simulink model "full_3omni_ctrl_sim_and_exp_with_bbb"  (R2019b)
settings: Solver=ode3  StartTime=0.0  StopTime=40  FixedStep=0.01  RelTol=1e-3  EnableMultiTasking=on
libraries: bbblueCommlib x24, simulink x10, bbblueSensorLib x4, xpcutilitieslib x3, xpcrtudplib x2, slrtlib x1
(part 1 of 2)
settings Model: SimulationMode=external  ExtModeTrigDuration=100  Creator=Sarot PC  LastModifiedBy=ONLY-GOD
settings SolverCC: PositivePriorityOrder=on
settings DataIOCC: SaveFormat=StructureWithTime
settings OptimizationCC: BlockReduction=off  EnhancedBackFolding=on  PassReuseOutputArgsAs=Individual arguments  ZeroExternalMemoryAtStartup=off  ZeroInternalMemoryAtStartup=off  MaxStackSize=64  OptimizeBlockOrder=speed  DifferentSizesBufferReuse=on  OptimizationCustomize=off  EfficientTunableParamExpr=on
settings DebuggingCC: ParameterTunabilityLossMsg=error  SFExecutionAtInitializationDiag=none  ArithmeticOperatorsInVariantConditions=warning
settings HardwareCC: ProdBitPerPointer=32  ProdBitPerSizeT=32  ProdBitPerPtrDiffT=32  ProdLargestAtomicInteger=Long  ProdLargestAtomicFloat=Double  ProdWordSize=32  ProdHWDeviceType=ARM Compatible->ARM Cortex
settings SFSimCC: MATLABDynamicMemAlloc=off  CustomCodeUndefinedFunction=UseInterfaceOnly
settings RTWCC: SystemTargetFile=ert.tlc  HardwareBoard=BeagleBone Blue  TLCOptions="-aInlineSetEventsForThisBaseRateFcn=TLC_FALSE -aSuppressMultiTaskScheduler=TLC_FALSE  -aRateBasedStepFcn=0"  TemplateMakefile=ert_default_tmf  GenerateReport=on  Toolchain=GNU GCC BeagleBone Blue  IncludeHyperlinkInReport=on  LaunchReport=on  GenerateTraceInfo=on  GenerateTraceReport=on  GenerateTraceReportSl=on  GenerateTraceReportSf=on  GenerateTraceReportEml=on
settings CodeAppCC: ForceParamTrailComments=on  IgnoreCustomStorageClasses=off  OperatorAnnotations=on  SimulinkDataObjDesc=on  SFDataObjDesc=on  InsertBlockDesc=on
settings ERTTargetCC: SupportContinuousTime=on  SupportVariableSizeSignals=on

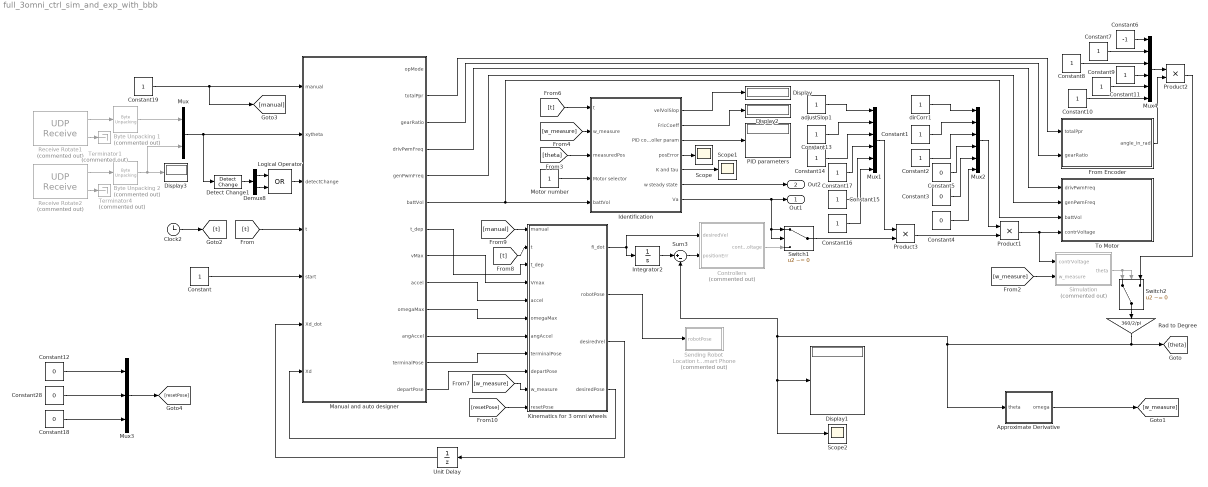
== system full_3omni_ctrl_sim_and_exp_with_bbb ==
  Approximate Derivative : Subsystem
  Byte Unpacking 1 : xpcutilitieslib/Byte Unpacking   Commented=on  MaskUnpackedDataTypes={'double'}  MaskUnpackedDataSizes={[1]}  MaskAlignment=1
      settings: SourceProductName=Simulink Real-Time  SourceProductBaseCode=XP
  Byte Unpacking 2 : xpcutilitieslib/Byte Unpacking   Commented=on  MaskUnpackedDataTypes={'double'}  MaskUnpackedDataSizes={[1]}  MaskAlignment=1
      settings: SourceProductName=Simulink Real-Time  SourceProductBaseCode=XP
  Clock2 : Clock
  Constant{,1..2,7..11,13..17,19} (14 alike) : Constant
  Constant{3..5,12,18,28} (6 alike) : Constant  Value=0
  Constant6 : Constant  Value=-1
  Controllers : Subsystem  Commented=on
  Demux8 : Demux  Outputs=2
  Detect Change1 : simulink/Logic and Bit Operations/Detect Change  vinit=0  OutDataTypeStr=boolean
  Display{,1..3} (4 alike) : Display
  From Encoder : Subsystem
  Identification : Subsystem
  Integrator2 : Integrator  InitialCondition=zeros(6,1)
  Kinematics for 3 omni wheels : Subsystem
  Logical Operator : Logic  Operator=OR  AllPortsSameDT=off  OutDataTypeStr=boolean
  Manual and auto designer : Stateflow chart  TreatAsAtomicUnit=on
  Motor number : Constant
  Mux : Mux  Inputs=2
  Mux1 : Mux  Inputs=6
  Mux2 : Mux  Inputs=6
  Mux3 : Mux  Inputs=3
  Mux4 : Mux  Inputs=6
  PID parameters : Display
  Product1 : Product
  Product2 : Product
  Product3 : Product
  Rad to Degree : Gain  Gain=360/2/pi
  Receive Rotate1 : xpcrtudplib/UDP Receive  Commented=on  ipAddressVal=Use host-target connection  localPort=2501  rcvWidth=8  rcvFmAny=off  fmAddress=192.168.88.233  rcvMulticast=off  multicastAddress={}  maxUDPQueue=8  sampleTime=-1
      settings: SourceProductName=Simulink Real-Time
  Receive Rotate2 : xpcrtudplib/UDP Receive  Commented=on  ipAddressVal=Use host-target connection  localPort=2502  rcvWidth=8  rcvFmAny=off  fmAddress=192.168.88.233  rcvMulticast=off  multicastAddress={}  maxUDPQueue=8  sampleTime=-1
      settings: SourceProductName=Simulink Real-Time
  Scope : Scope
  Scope1 : Scope
  Scope2 : Scope
  Sending Robot Location to Smart Phone : Subsystem  Commented=on
  Simulation : Subsystem  Commented=on
  Sum3 : Sum  Inputs=|+-
  Switch1 : Switch  Criteria=u2 ~= 0
  Switch2 : Switch  Criteria=u2 ~= 0
  Terminator1 : Terminator  Commented=on
  Terminator4 : Terminator  Commented=on
  To Motor : Subsystem
  Unit Delay : UnitDelay  InitialCondition=[0;0;0]  SampleTime=-1  HasFrameUpgradeWarning=on
  adjustSlop1 : Constant
  dirCorr1 : Constant
  Out1 : Outport
  Out2 : Outport  Port=2
  wires:
  Constant2/1 -> Mux2/3
  dirCorr1/1 -> Mux2/1
  Constant1/1 -> Mux2/2
  Mux2/1 -> Product1/1
  Product1/1 -> Simulation/1(contrVoltage), To Motor/4(contrVoltage)
  Product3/1 -> Product1/2
  Constant5/1 -> Mux2/4
  Constant3/1 -> Mux2/5
  Constant4/1 -> Mux2/6
  Constant10/1 -> Mux4/6
  Constant6/1 -> Mux4/1
  Constant7/1 -> Mux4/2
  Mux4/1 -> Product2/1
  Constant11/1 -> Mux4/4
  Constant9/1 -> Mux4/5
  Constant8/1 -> Mux4/3
  From Encoder/1(angle_in_rad) -> Product2/2
  Product2/1 -> Switch2/3
  Constant16/1 -> Mux1/6
  Constant15/1 -> Mux1/5
  Constant17/1 -> Mux1/4
  Mux1/1 -> Product3/1
  Constant13/1 -> Mux1/2
  adjustSlop1/1 -> Mux1/1
  Constant14/1 -> Mux1/3
  Switch1/1 -> Product3/2
  Manual and auto designer/2(totalPpr) -> From Encoder/1(totalPpr)
  Manual and auto designer/3(gearRatio) -> From Encoder/2(gearRatio)
  Simulation/1(theta) -> Switch2/2, Switch2/1
  Controllers/1(contrVoltage) -> Switch1/3
  Sum3/1 -> Controllers/2(positionErr)
  Identification/7(Va) -> Out1/1, Switch1/2, Switch1/1
  [t] -> Identification/1(t)
  [w_measure] -> Identification/2(w_measure)
  [theta] -> Identification/3(measuredPos)
  Identification/1(velVolSlop) -> Display/1
  Identification/3(PID controller param) -> PID parameters/1
  Identification/6(w steady state) -> Out2/1
  Identification/4(posError) -> Scope/1
  Identification/5(K and tau) -> Scope1/1
  Motor number/1 -> Identification/4(Motor selector)
  Integrator2/1 -> Sum3/1
  Kinematics for 3 omni wheels/1(fi_dot) -> Integrator2/1, Controllers/1(desiredVel)
  Manual and auto designer/4(drivPwmFreq) -> To Motor/1(drivPwmFreq)
  Manual and auto designer/5(genPwmFreq) -> To Motor/2(genPwmFreq)
  Manual and auto designer/6(battVol) -> To Motor/3(battVol), Identification/5(battVol)
  Identification/2(FricCoeff) -> Display2/1
  [w_measure] -> Simulation/2(w_measure)
  Demux8/2 -> Logical Operator/2
  Logical Operator/1 -> Manual and auto designer/3(detectChange)
  Mux/1 -> Detect Change1/1, Manual and auto designer/2(xytheta)
  Detect Change1/1 -> Demux8/1
  Kinematics for 3 omni wheels/4(desiredPose) -> Manual and auto designer/7(Xd)
  [t] -> Manual and auto designer/4(t)
  Constant/1 -> Manual and auto designer/5(start)
  Demux8/1 -> Logical Operator/1
  Constant19/1 -> [manual], Manual and auto designer/1(manual)
  Clock2/1 -> [t]
  [t] -> Kinematics for 3 omni wheels/2(t)
  Kinematics for 3 omni wheels/2(robotPose) -> Sending Robot Location to Smart Phone/1(robotPose)
  [w_measure] -> Kinematics for 3 omni wheels/10(w_measure)
  Kinematics for 3 omni wheels/3(desiredVel) -> Unit Delay/1
  Manual and auto designer/13(departPose) -> Kinematics for 3 omni wheels/9(departPose)
  Manual and auto designer/12(terminalPose) -> Kinematics for 3 omni wheels/8(terminalPose)
  Manual and auto designer/10(omegaMax) -> Kinematics for 3 omni wheels/6(omegaMax)
  Manual and auto designer/11(angAccel) -> Kinematics for 3 omni wheels/7(angAccel)
  Manual and auto designer/9(accel) -> Kinematics for 3 omni wheels/5(accel)
  Manual and auto designer/8(vMax) -> Kinematics for 3 omni wheels/4(Vmax)
  Manual and auto designer/7(t_dep) -> Kinematics for 3 omni wheels/3(t_dep)
  [manual] -> Kinematics for 3 omni wheels/1(manual)
  Unit Delay/1 -> Manual and auto designer/6(Xd_dot)
  Constant12/1 -> Mux3/1
  Constant28/1 -> Mux3/2
  Constant18/1 -> Mux3/3
  Mux3/1 -> [resetPose]
  [resetPose] -> Kinematics for 3 omni wheels/11(resetPose)
  Receive Rotate2/1 -> Byte Unpacking 2/1
  Receive Rotate1/2 -> Terminator1/1
  Byte Unpacking 1/1 -> Mux/1
  Receive Rotate2/2 -> Terminator4/1
  Receive Rotate1/1 -> Byte Unpacking 1/1
  Byte Unpacking 2/1 -> Mux/2, Display3/1
  Rad to Degree/1 -> [theta], Sum3/2, Scope2/1, Display1/1, Approximate Derivative/1(theta)
  Approximate Derivative/1(omega) -> [w_measure]
  Switch2/1 -> Rad to Degree/1

== system full_3omni_ctrl_sim_and_exp_with_bbb/Approximate Derivative ==
  theta : Inport
  Demux7 : Demux  Outputs=6
  Mux3 : Mux  Inputs=6
  Transfer Fcn{,1..5} (6 alike) : TransferFcn  Numerator=[1 0]  Denominator=[0.04 1]
  omega : Outport
  wires:
  Transfer Fcn1/1 -> Mux3/2
  Demux7/5 -> Transfer Fcn4/1
  Transfer Fcn3/1 -> Mux3/4
  Demux7/3 -> Transfer Fcn2/1
  Demux7/6 -> Transfer Fcn5/1
  Transfer Fcn2/1 -> Mux3/3
  Transfer Fcn/1 -> Mux3/1
  Transfer Fcn5/1 -> Mux3/6
  Demux7/4 -> Transfer Fcn3/1
  Mux3/1 -> omega/1
  Transfer Fcn4/1 -> Mux3/5
  Demux7/1 -> Transfer Fcn/1
  Demux7/2 -> Transfer Fcn1/1
  theta/1 -> Demux7/1

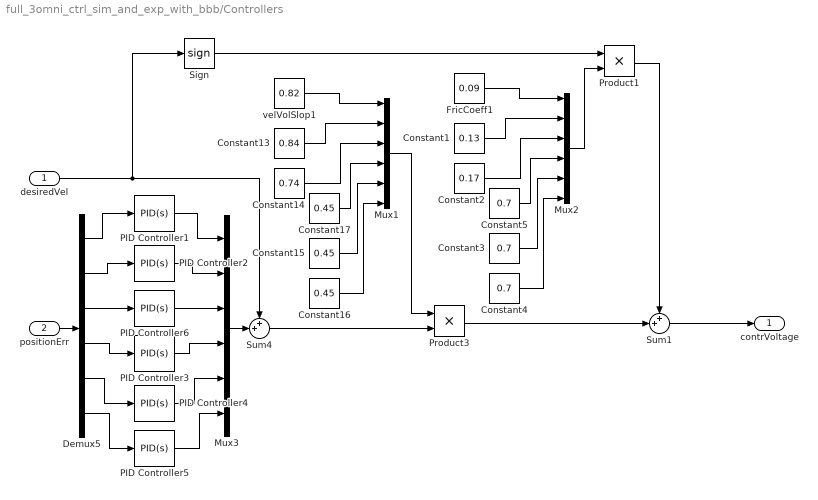
== system full_3omni_ctrl_sim_and_exp_with_bbb/Controllers ==
  desiredVel : Inport
  positionErr : Inport  Port=2
  Constant1 : Constant  Value=0.13
  Constant13 : Constant  Value=0.84
  Constant14 : Constant  Value=0.74
  Constant15 : Constant  Value=0.45
  Constant16 : Constant  Value=0.45
  Constant17 : Constant  Value=0.45
  Constant2 : Constant  Value=0.17
  Constant3 : Constant  Value=0.7
  Constant4 : Constant  Value=0.7
  Constant5 : Constant  Value=0.7
  Demux5 : Demux  Outputs=6
  FricCoeff1 : Constant  Value=0.09
  Mux1 : Mux  Inputs=6
  Mux2 : Mux  Inputs=6
  Mux3 : Mux  Inputs=6
  "PID Controller1 " : simulink/Continuous/PID Controller  Controller=PID  Form=Parallel  TimeDomain=Continuous-time  SampleTime=-1  IntegratorMethod=Forward Euler  FilterMethod=Forward Euler  ControllerParametersSource=internal  P=45/0.82  I=0  D=2.9/0.82  UseFilter=on  N=100  TunerSelectOption=Transfer Function Based (PID Tuner App)  InitialConditionSource=internal  InitialConditionForIntegrator=0  InitialConditionForFilter=0  DifferentiatorICPrevScaledInput=0  ExternalReset=none  TrackingMode=off  Kt=1  LimitOutput=off  UpperSaturationLimit=inf  LowerSaturationLimit=-inf  LinearizeAsGain=on  AntiWindupMode=none  Kb=1  POutMin=[]  POutMax=[]  IOutMin=[]  IOutMax=[]  DOutMin=[]  DOutMax=[]  NOutMin=[]  NOutMax=[]  SumOutMin=[]  SumOutMax=[]  SaturationOutMin=[]  SaturationOutMax=[]  PParamMin=[]  PParamMax=[]  IParamMin=[]  IParamMax=[]  DParamMin=[]  DParamMax=[]  NParamMin=[]  NParamMax=[]  KbParamMin=[]  KbParamMax=[]  KtParamMin=[]  KtParamMax=[]  KbOutMin=[]  KbOutMax=[]  KtOutMin=[]  KtOutMax=[]  IntegratorOutMin=[]  IntegratorOutMax=[]  FilterOutMin=[]  FilterOutMax=[]  SumI1OutMin=[]  SumI1OutMax=[]  SumI2OutMin=[]  SumI2OutMax=[]  SumI3OutMin=[]  SumI3OutMax=[]  SumI4OutMin=[]  SumI4OutMax=[]  SumDOutMin=[]  SumDOutMax=[]  DifferentiatorOutMin=[]  DifferentiatorOutMax=[]  FilterDiffOutCoefMin=[]  FilterDiffOutCoefMax=[]  ReciprocalOutMin=[]  ReciprocalOutMax=[]  SumDenOutMin=[]  SumDenOutMax=[]  SumNumOutMin=[]  SumNumOutMax=[]  DivideOutMin=[]  DivideOutMax=[]  IntegratorContinuousStateAttributes=''  IntegratorStateMustResolveToSignalObject=off  IntegratorRTWStateStorageClass=Auto  FilterContinuousStateAttributes=''  FilterStateMustResolveToSignalObject=off  FilterRTWStateStorageClass=Auto  ParallelPVariant=InternalParameters  IdealPVariant=Disabled  IVariant=InternalParameters  DVariant=InternalParameters  IntegratorVariant=Continuous  SatVariant=Disabled  AWVariant=Passthrough  PCopyVariant=Disabled  TRVariant=Disabled  FdbkBlocksVariant=Forward  IdealPFdbkVariant=Disabled  SatFdbkVariant=Disabled  DerivativeFilterVariant=ContFilter  NVariant=InternalParameters  NCopyVariant=Disabled  FilterICVariant=InternalICsFilter  IntegratorICVariant=InternalICs  ExternalResetVariant=Disabled  TRSumVariant=Passthrough  SumFdbkVariant=Disabled  SumVariant=Sum_PID
  PID Controller2 : simulink/Continuous/PID Controller  Controller=PID  Form=Parallel  TimeDomain=Continuous-time  SampleTime=-1  IntegratorMethod=Forward Euler  FilterMethod=Forward Euler  ControllerParametersSource=internal  P=45/0.84  I=0  D=2.96/0.84  UseFilter=on  N=100  TunerSelectOption=Transfer Function Based (PID Tuner App)  InitialConditionSource=internal  InitialConditionForIntegrator=0  InitialConditionForFilter=0  DifferentiatorICPrevScaledInput=0  ExternalReset=none  TrackingMode=off  Kt=1  LimitOutput=off  UpperSaturationLimit=inf  LowerSaturationLimit=-inf  LinearizeAsGain=on  AntiWindupMode=none  Kb=1  POutMin=[]  POutMax=[]  IOutMin=[]  IOutMax=[]  DOutMin=[]  DOutMax=[]  NOutMin=[]  NOutMax=[]  SumOutMin=[]  SumOutMax=[]  SaturationOutMin=[]  SaturationOutMax=[]  PParamMin=[]  PParamMax=[]  IParamMin=[]  IParamMax=[]  DParamMin=[]  DParamMax=[]  NParamMin=[]  NParamMax=[]  KbParamMin=[]  KbParamMax=[]  KtParamMin=[]  KtParamMax=[]  KbOutMin=[]  KbOutMax=[]  KtOutMin=[]  KtOutMax=[]  IntegratorOutMin=[]  IntegratorOutMax=[]  FilterOutMin=[]  FilterOutMax=[]  SumI1OutMin=[]  SumI1OutMax=[]  SumI2OutMin=[]  SumI2OutMax=[]  SumI3OutMin=[]  SumI3OutMax=[]  SumI4OutMin=[]  SumI4OutMax=[]  SumDOutMin=[]  SumDOutMax=[]  DifferentiatorOutMin=[]  DifferentiatorOutMax=[]  FilterDiffOutCoefMin=[]  FilterDiffOutCoefMax=[]  ReciprocalOutMin=[]  ReciprocalOutMax=[]  SumDenOutMin=[]  SumDenOutMax=[]  SumNumOutMin=[]  SumNumOutMax=[]  DivideOutMin=[]  DivideOutMax=[]  IntegratorContinuousStateAttributes=''  IntegratorStateMustResolveToSignalObject=off  IntegratorRTWStateStorageClass=Auto  FilterContinuousStateAttributes=''  FilterStateMustResolveToSignalObject=off  FilterRTWStateStorageClass=Auto  ParallelPVariant=InternalParameters  IdealPVariant=Disabled  IVariant=InternalParameters  DVariant=InternalParameters  IntegratorVariant=Continuous  SatVariant=Disabled  AWVariant=Passthrough  PCopyVariant=Disabled  TRVariant=Disabled  FdbkBlocksVariant=Forward  IdealPFdbkVariant=Disabled  SatFdbkVariant=Disabled  DerivativeFilterVariant=ContFilter  NVariant=InternalParameters  NCopyVariant=Disabled  FilterICVariant=InternalICsFilter  IntegratorICVariant=InternalICs  ExternalResetVariant=Disabled  TRSumVariant=Passthrough  SumFdbkVariant=Disabled  SumVariant=Sum_PID
  PID Controller3 : simulink/Continuous/PID Controller  Controller=PID  Form=Parallel  TimeDomain=Continuous-time  SampleTime=-1  IntegratorMethod=Forward Euler  FilterMethod=Forward Euler  ControllerParametersSource=internal  P=10  I=0  D=3  UseFilter=on  N=100  TunerSelectOption=Transfer Function Based (PID Tuner App)  InitialConditionSource=internal  InitialConditionForIntegrator=0  InitialConditionForFilter=0  DifferentiatorICPrevScaledInput=0  ExternalReset=none  TrackingMode=off  Kt=1  LimitOutput=off  UpperSaturationLimit=inf  LowerSaturationLimit=-inf  LinearizeAsGain=on  AntiWindupMode=none  Kb=1  POutMin=[]  POutMax=[]  IOutMin=[]  IOutMax=[]  DOutMin=[]  DOutMax=[]  NOutMin=[]  NOutMax=[]  SumOutMin=[]  SumOutMax=[]  SaturationOutMin=[]  SaturationOutMax=[]  PParamMin=[]  PParamMax=[]  IParamMin=[]  IParamMax=[]  DParamMin=[]  DParamMax=[]  NParamMin=[]  NParamMax=[]  KbParamMin=[]  KbParamMax=[]  KtParamMin=[]  KtParamMax=[]  KbOutMin=[]  KbOutMax=[]  KtOutMin=[]  KtOutMax=[]  IntegratorOutMin=[]  IntegratorOutMax=[]  FilterOutMin=[]  FilterOutMax=[]  SumI1OutMin=[]  SumI1OutMax=[]  SumI2OutMin=[]  SumI2OutMax=[]  SumI3OutMin=[]  SumI3OutMax=[]  SumI4OutMin=[]  SumI4OutMax=[]  SumDOutMin=[]  SumDOutMax=[]  DifferentiatorOutMin=[]  DifferentiatorOutMax=[]  FilterDiffOutCoefMin=[]  FilterDiffOutCoefMax=[]  ReciprocalOutMin=[]  ReciprocalOutMax=[]  SumDenOutMin=[]  SumDenOutMax=[]  SumNumOutMin=[]  SumNumOutMax=[]  DivideOutMin=[]  DivideOutMax=[]  IntegratorContinuousStateAttributes=''  IntegratorStateMustResolveToSignalObject=off  IntegratorRTWStateStorageClass=Auto  FilterContinuousStateAttributes=''  FilterStateMustResolveToSignalObject=off  FilterRTWStateStorageClass=Auto  ParallelPVariant=InternalParameters  IdealPVariant=Disabled  IVariant=InternalParameters  DVariant=InternalParameters  IntegratorVariant=Continuous  SatVariant=Disabled  AWVariant=Passthrough  PCopyVariant=Disabled  TRVariant=Disabled  FdbkBlocksVariant=Forward  IdealPFdbkVariant=Disabled  SatFdbkVariant=Disabled  DerivativeFilterVariant=ContFilter  NVariant=InternalParameters  NCopyVariant=Disabled  FilterICVariant=InternalICsFilter  IntegratorICVariant=InternalICs  ExternalResetVariant=Disabled  TRSumVariant=Passthrough  SumFdbkVariant=Disabled  SumVariant=Sum_PID
  PID Controller4 : simulink/Continuous/PID Controller  Controller=PID  Form=Parallel  TimeDomain=Continuous-time  SampleTime=-1  IntegratorMethod=Forward Euler  FilterMethod=Forward Euler  ControllerParametersSource=internal  P=10  I=0  D=3  UseFilter=on  N=100  TunerSelectOption=Transfer Function Based (PID Tuner App)  InitialConditionSource=internal  InitialConditionForIntegrator=0  InitialConditionForFilter=0  DifferentiatorICPrevScaledInput=0  ExternalReset=none  TrackingMode=off  Kt=1  LimitOutput=off  UpperSaturationLimit=inf  LowerSaturationLimit=-inf  LinearizeAsGain=on  AntiWindupMode=none  Kb=1  POutMin=[]  POutMax=[]  IOutMin=[]  IOutMax=[]  DOutMin=[]  DOutMax=[]  NOutMin=[]  NOutMax=[]  SumOutMin=[]  SumOutMax=[]  SaturationOutMin=[]  SaturationOutMax=[]  PParamMin=[]  PParamMax=[]  IParamMin=[]  IParamMax=[]  DParamMin=[]  DParamMax=[]  NParamMin=[]  NParamMax=[]  KbParamMin=[]  KbParamMax=[]  KtParamMin=[]  KtParamMax=[]  KbOutMin=[]  KbOutMax=[]  KtOutMin=[]  KtOutMax=[]  IntegratorOutMin=[]  IntegratorOutMax=[]  FilterOutMin=[]  FilterOutMax=[]  SumI1OutMin=[]  SumI1OutMax=[]  SumI2OutMin=[]  SumI2OutMax=[]  SumI3OutMin=[]  SumI3OutMax=[]  SumI4OutMin=[]  SumI4OutMax=[]  SumDOutMin=[]  SumDOutMax=[]  DifferentiatorOutMin=[]  DifferentiatorOutMax=[]  FilterDiffOutCoefMin=[]  FilterDiffOutCoefMax=[]  ReciprocalOutMin=[]  ReciprocalOutMax=[]  SumDenOutMin=[]  SumDenOutMax=[]  SumNumOutMin=[]  SumNumOutMax=[]  DivideOutMin=[]  DivideOutMax=[]  IntegratorContinuousStateAttributes=''  IntegratorStateMustResolveToSignalObject=off  IntegratorRTWStateStorageClass=Auto  FilterContinuousStateAttributes=''  FilterStateMustResolveToSignalObject=off  FilterRTWStateStorageClass=Auto  ParallelPVariant=InternalParameters  IdealPVariant=Disabled  IVariant=InternalParameters  DVariant=InternalParameters  IntegratorVariant=Continuous  SatVariant=Disabled  AWVariant=Passthrough  PCopyVariant=Disabled  TRVariant=Disabled  FdbkBlocksVariant=Forward  IdealPFdbkVariant=Disabled  SatFdbkVariant=Disabled  DerivativeFilterVariant=ContFilter  NVariant=InternalParameters  NCopyVariant=Disabled  FilterICVariant=InternalICsFilter  IntegratorICVariant=InternalICs  ExternalResetVariant=Disabled  TRSumVariant=Passthrough  SumFdbkVariant=Disabled  SumVariant=Sum_PID
  PID Controller5 : simulink/Continuous/PID Controller  Controller=PID  Form=Parallel  TimeDomain=Continuous-time  SampleTime=-1  IntegratorMethod=Forward Euler  FilterMethod=Forward Euler  ControllerParametersSource=internal  P=10  I=0  D=3  UseFilter=on  N=100  TunerSelectOption=Transfer Function Based (PID Tuner App)  InitialConditionSource=internal  InitialConditionForIntegrator=0  InitialConditionForFilter=0  DifferentiatorICPrevScaledInput=0  ExternalReset=none  TrackingMode=off  Kt=1  LimitOutput=off  UpperSaturationLimit=inf  LowerSaturationLimit=-inf  LinearizeAsGain=on  AntiWindupMode=none  Kb=1  POutMin=[]  POutMax=[]  IOutMin=[]  IOutMax=[]  DOutMin=[]  DOutMax=[]  NOutMin=[]  NOutMax=[]  SumOutMin=[]  SumOutMax=[]  SaturationOutMin=[]  SaturationOutMax=[]  PParamMin=[]  PParamMax=[]  IParamMin=[]  IParamMax=[]  DParamMin=[]  DParamMax=[]  NParamMin=[]  NParamMax=[]  KbParamMin=[]  KbParamMax=[]  KtParamMin=[]  KtParamMax=[]  KbOutMin=[]  KbOutMax=[]  KtOutMin=[]  KtOutMax=[]  IntegratorOutMin=[]  IntegratorOutMax=[]  FilterOutMin=[]  FilterOutMax=[]  SumI1OutMin=[]  SumI1OutMax=[]  SumI2OutMin=[]  SumI2OutMax=[]  SumI3OutMin=[]  SumI3OutMax=[]  SumI4OutMin=[]  SumI4OutMax=[]  SumDOutMin=[]  SumDOutMax=[]  DifferentiatorOutMin=[]  DifferentiatorOutMax=[]  FilterDiffOutCoefMin=[]  FilterDiffOutCoefMax=[]  ReciprocalOutMin=[]  ReciprocalOutMax=[]  SumDenOutMin=[]  SumDenOutMax=[]  SumNumOutMin=[]  SumNumOutMax=[]  DivideOutMin=[]  DivideOutMax=[]  IntegratorContinuousStateAttributes=''  IntegratorStateMustResolveToSignalObject=off  IntegratorRTWStateStorageClass=Auto  FilterContinuousStateAttributes=''  FilterStateMustResolveToSignalObject=off  FilterRTWStateStorageClass=Auto  ParallelPVariant=InternalParameters  IdealPVariant=Disabled  IVariant=InternalParameters  DVariant=InternalParameters  IntegratorVariant=Continuous  SatVariant=Disabled  AWVariant=Passthrough  PCopyVariant=Disabled  TRVariant=Disabled  FdbkBlocksVariant=Forward  IdealPFdbkVariant=Disabled  SatFdbkVariant=Disabled  DerivativeFilterVariant=ContFilter  NVariant=InternalParameters  NCopyVariant=Disabled  FilterICVariant=InternalICsFilter  IntegratorICVariant=InternalICs  ExternalResetVariant=Disabled  TRSumVariant=Passthrough  SumFdbkVariant=Disabled  SumVariant=Sum_PID
  PID Controller6 : simulink/Continuous/PID Controller  Controller=PID  Form=Parallel  TimeDomain=Continuous-time  SampleTime=-1  IntegratorMethod=Forward Euler  FilterMethod=Forward Euler  ControllerParametersSource=internal  P=45/0.74  I=0  D=2.59/0.74  UseFilter=on  N=100  TunerSelectOption=Transfer Function Based (PID Tuner App)  InitialConditionSource=internal  InitialConditionForIntegrator=0  InitialConditionForFilter=0  DifferentiatorICPrevScaledInput=0  ExternalReset=none  TrackingMode=off  Kt=1  LimitOutput=off  UpperSaturationLimit=inf  LowerSaturationLimit=-inf  LinearizeAsGain=on  AntiWindupMode=none  Kb=1  POutMin=[]  POutMax=[]  IOutMin=[]  IOutMax=[]  DOutMin=[]  DOutMax=[]  NOutMin=[]  NOutMax=[]  SumOutMin=[]  SumOutMax=[]  SaturationOutMin=[]  SaturationOutMax=[]  PParamMin=[]  PParamMax=[]  IParamMin=[]  IParamMax=[]  DParamMin=[]  DParamMax=[]  NParamMin=[]  NParamMax=[]  KbParamMin=[]  KbParamMax=[]  KtParamMin=[]  KtParamMax=[]  KbOutMin=[]  KbOutMax=[]  KtOutMin=[]  KtOutMax=[]  IntegratorOutMin=[]  IntegratorOutMax=[]  FilterOutMin=[]  FilterOutMax=[]  SumI1OutMin=[]  SumI1OutMax=[]  SumI2OutMin=[]  SumI2OutMax=[]  SumI3OutMin=[]  SumI3OutMax=[]  SumI4OutMin=[]  SumI4OutMax=[]  SumDOutMin=[]  SumDOutMax=[]  DifferentiatorOutMin=[]  DifferentiatorOutMax=[]  FilterDiffOutCoefMin=[]  FilterDiffOutCoefMax=[]  ReciprocalOutMin=[]  ReciprocalOutMax=[]  SumDenOutMin=[]  SumDenOutMax=[]  SumNumOutMin=[]  SumNumOutMax=[]  DivideOutMin=[]  DivideOutMax=[]  IntegratorContinuousStateAttributes=''  IntegratorStateMustResolveToSignalObject=off  IntegratorRTWStateStorageClass=Auto  FilterContinuousStateAttributes=''  FilterStateMustResolveToSignalObject=off  FilterRTWStateStorageClass=Auto  ParallelPVariant=InternalParameters  IdealPVariant=Disabled  IVariant=InternalParameters  DVariant=InternalParameters  IntegratorVariant=Continuous  SatVariant=Disabled  AWVariant=Passthrough  PCopyVariant=Disabled  TRVariant=Disabled  FdbkBlocksVariant=Forward  IdealPFdbkVariant=Disabled  SatFdbkVariant=Disabled  DerivativeFilterVariant=ContFilter  NVariant=InternalParameters  NCopyVariant=Disabled  FilterICVariant=InternalICsFilter  IntegratorICVariant=InternalICs  ExternalResetVariant=Disabled  TRSumVariant=Passthrough  SumFdbkVariant=Disabled  SumVariant=Sum_PID
  Product1 : Product
  Product3 : Product
  Sign : Signum
  Sum1 : Sum  Inputs=++|
  Sum4 : Sum  Inputs=++|
  velVolSlop1 : Constant  Value=0.82
  contrVoltage : Outport
  wires:
  PID Controller2/1 -> Mux3/2
  Demux5/3 -> PID Controller6/1
  Demux5/1 -> "PID Controller1 "/1
  PID Controller6/1 -> Mux3/3
  "PID Controller1 "/1 -> Mux3/1
  positionErr/1 -> Demux5/1
  Demux5/2 -> PID Controller2/1
  Demux5/4 -> PID Controller3/1
  Demux5/5 -> PID Controller4/1
  Demux5/6 -> PID Controller5/1
  PID Controller3/1 -> Mux3/4
  PID Controller4/1 -> Mux3/5
  PID Controller5/1 -> Mux3/6
  Constant16/1 -> Mux1/6
  Constant15/1 -> Mux1/5
  Constant14/1 -> Mux1/3
  Constant13/1 -> Mux1/2
  velVolSlop1/1 -> Mux1/1
  Mux1/1 -> Product3/1
  Constant17/1 -> Mux1/4
  Sum1/1 -> contrVoltage/1
  Mux3/1 -> Sum4/2
  Sum4/1 -> Product3/2
  desiredVel/1 -> Sign/1, Sum4/1
  Product3/1 -> Sum1/2
  Constant2/1 -> Mux2/3
  Constant5/1 -> Mux2/4
  FricCoeff1/1 -> Mux2/1
  Constant4/1 -> Mux2/6
  Constant3/1 -> Mux2/5
  Constant1/1 -> Mux2/2
  Sign/1 -> Product1/1
  Mux2/1 -> Product1/2
  Product1/1 -> Sum1/1

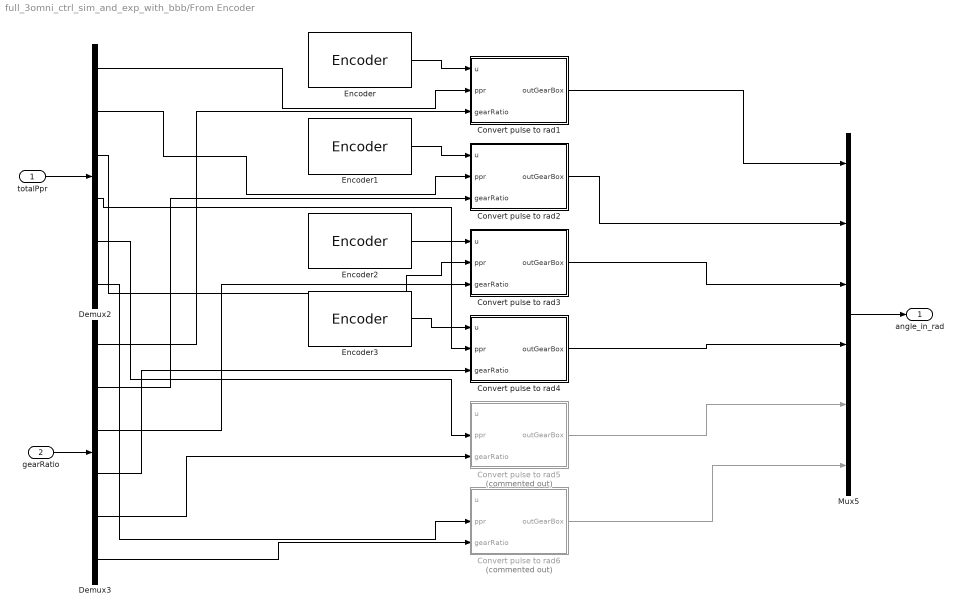
== system full_3omni_ctrl_sim_and_exp_with_bbb/From Encoder ==
  totalPpr : Inport
  gearRatio : Inport  Port=2
  Convert pulse to rad1 : MATLAB Function  TreatAsAtomicUnit=on
  Convert pulse to rad2 : MATLAB Function  TreatAsAtomicUnit=on
  Convert pulse to rad3 : MATLAB Function  TreatAsAtomicUnit=on
  Convert pulse to rad4 : MATLAB Function  TreatAsAtomicUnit=on
  Convert pulse to rad5 : MATLAB Function  Commented=on  TreatAsAtomicUnit=on
  Convert pulse to rad6 : MATLAB Function  Commented=on  TreatAsAtomicUnit=on
  Demux2 : Demux  Outputs=6
  Demux3 : Demux  Outputs=6
  Encoder : bbblueSensorLib/Encoder  Channel=1  Mode=No reset  SampleTime=0.01  SimulateUsing=Code generation
      settings: SourceProductName=Simulink Coder Support Package for BeagleBone Blue Hardware  SourceProductBaseCode=SC_BEAGLEBONE_BLUE
  Encoder1 : bbblueSensorLib/Encoder  Channel=2  Mode=No reset  SampleTime=0.01  SimulateUsing=Code generation
      settings: SourceProductName=Simulink Coder Support Package for BeagleBone Blue Hardware  SourceProductBaseCode=SC_BEAGLEBONE_BLUE
  Encoder2 : bbblueSensorLib/Encoder  Channel=3  Mode=No reset  SampleTime=0.01  SimulateUsing=Code generation
      settings: SourceProductName=Simulink Coder Support Package for BeagleBone Blue Hardware  SourceProductBaseCode=SC_BEAGLEBONE_BLUE
  Encoder3 : bbblueSensorLib/Encoder  Channel=4  Mode=No reset  SampleTime=0.01  SimulateUsing=Code generation
      settings: SourceProductName=Simulink Coder Support Package for BeagleBone Blue Hardware  SourceProductBaseCode=SC_BEAGLEBONE_BLUE
  Mux5 : Mux  Inputs=6
  angle_in_rad : Outport
  wires:
  Demux3/5 -> Convert pulse to rad5/3(gearRatio)
  Demux3/6 -> Convert pulse to rad6/3(gearRatio)
  Demux3/1 -> Convert pulse to rad1/3(gearRatio)
  Convert pulse to rad3/1(outGearBox) -> Mux5/3
  Convert pulse to rad5/1(outGearBox) -> Mux5/5
  Mux5/1 -> angle_in_rad/1
  Demux2/2 -> Convert pulse to rad2/2(ppr)
  gearRatio/1 -> Demux3/1
  ? -> Convert pulse to rad5/1(u)
  Demux2/5 -> Convert pulse to rad5/2(ppr)
  Encoder3/1 -> Convert pulse to rad4/1(u)
  Demux2/6 -> Convert pulse to rad6/2(ppr)
  Demux2/3 -> Convert pulse to rad3/2(ppr)
  Demux3/3 -> Convert pulse to rad3/3(gearRatio)
  Encoder1/1 -> Convert pulse to rad2/1(u)
  Demux2/4 -> Convert pulse to rad4/2(ppr)
  Demux2/1 -> Convert pulse to rad1/2(ppr)
  Convert pulse to rad6/1(outGearBox) -> Mux5/6
  Demux3/4 -> Convert pulse to rad4/3(gearRatio)
  Convert pulse to rad1/1(outGearBox) -> Mux5/1
  Encoder2/1 -> Convert pulse to rad3/1(u)
  Convert pulse to rad4/1(outGearBox) -> Mux5/4
  Demux3/2 -> Convert pulse to rad2/3(gearRatio)
  Convert pulse to rad2/1(outGearBox) -> Mux5/2
  totalPpr/1 -> Demux2/1
  ? -> Convert pulse to rad6/1(u)
  Encoder/1 -> Convert pulse to rad1/1(u)

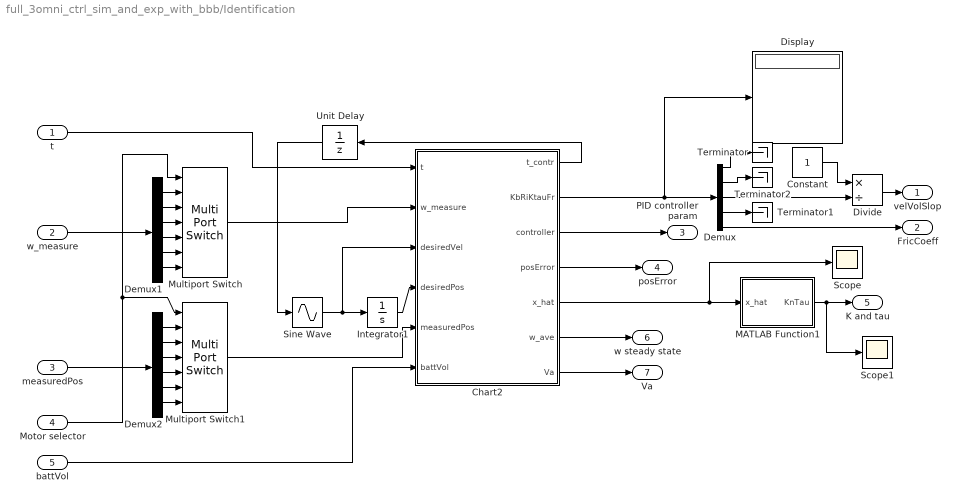
== system full_3omni_ctrl_sim_and_exp_with_bbb/Identification ==
  t : Inport
  w_measure : Inport  Port=2
  measuredPos : Inport  Port=3
  Motor selector : Inport  Port=4
  battVol : Inport  Port=5
  Chart2 : Stateflow chart  TreatAsAtomicUnit=on
  Constant : Constant
  Demux : Demux  Outputs=5
  Demux1 : Demux  Outputs=6
  Demux2 : Demux  Outputs=6
  Display : Display
  Divide : Product  Inputs=*/
  Integrator1 : Integrator
  MATLAB Function1 : MATLAB Function  TreatAsAtomicUnit=on
  Multiport Switch : MultiPortSwitch  Inputs=6
  Multiport Switch1 : MultiPortSwitch  Inputs=6
  Scope : Scope
  Scope1 : Scope
  Sine Wave : Sin  TimeSource=Use external signal  Amplitude=pi  SampleTime=0
  Terminator : Terminator
  Terminator1 : Terminator
  Terminator2 : Terminator
  Unit Delay : UnitDelay  SampleTime=-1  HasFrameUpgradeWarning=on
  velVolSlop : Outport
  FricCoeff : Outport  Port=2
  PID controller param : Outport  Port=3
  posError : Outport  Port=4
  K and tau : Outport  Port=5
  w steady state : Outport  Port=6
  Va : Outport  Port=7
  wires:
  Sine Wave/1 -> Chart2/3(desiredVel), Integrator1/1
  Chart2/5(x_hat) -> Scope/1, MATLAB Function1/1(x_hat)
  Multiport Switch/1 -> Chart2/2(w_measure)
  Chart2/7(Va) -> Va/1
  Chart2/1(t_contr) -> Unit Delay/1
  Integrator1/1 -> Chart2/4(desiredPos)
  Unit Delay/1 -> Sine Wave/1
  Chart2/4(posError) -> posError/1
  MATLAB Function1/1(KnTau) -> Scope1/1, K and tau/1
  Multiport Switch1/1 -> Chart2/5(measuredPos)
  t/1 -> Chart2/1(t)
  Chart2/2(KbRiKtauFr) -> Display/1, Demux/1
  Chart2/3(controller) -> PID controller param/1
  Chart2/6(w_ave) -> w steady state/1
  Demux/3 -> Divide/2
  Divide/1 -> velVolSlop/1
  Constant/1 -> Divide/1
  Demux/1 -> Terminator/1
  Demux/4 -> Terminator1/1
  Demux/2 -> Terminator2/1
  Demux1/1 -> Multiport Switch/2
  Demux1/2 -> Multiport Switch/3
  Demux1/3 -> Multiport Switch/4
  Demux1/4 -> Multiport Switch/5
  Demux1/5 -> Multiport Switch/6
  Demux1/6 -> Multiport Switch/7
  Demux2/1 -> Multiport Switch1/2
  Demux2/2 -> Multiport Switch1/3
  Demux2/3 -> Multiport Switch1/4
  Demux2/4 -> Multiport Switch1/5
  Demux2/5 -> Multiport Switch1/6
  Demux2/6 -> Multiport Switch1/7
  measuredPos/1 -> Demux2/1
  w_measure/1 -> Demux1/1
  Motor selector/1 -> Multiport Switch1/1, Multiport Switch/1
  Demux/5 -> FricCoeff/1
  battVol/1 -> Chart2/6(battVol)

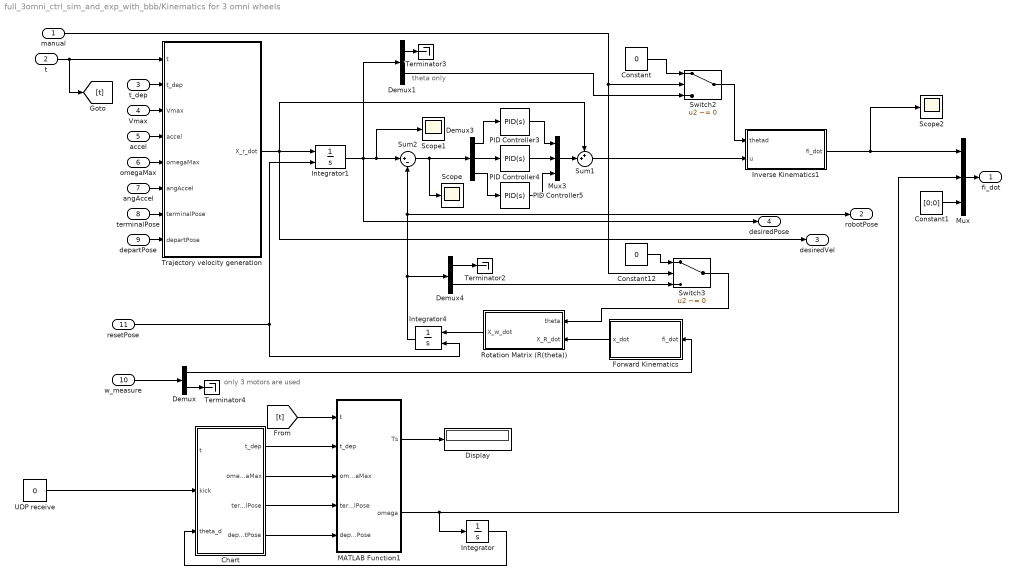
== system full_3omni_ctrl_sim_and_exp_with_bbb/Kinematics for 3 omni wheels ==
  note: only 3 motors are used
  note: theta only
  manual : Inport
  t : Inport  Port=2
  t_dep : Inport  Port=3
  Vmax : Inport  Port=4
  accel : Inport  Port=5
  omegaMax : Inport  Port=6
  angAccel : Inport  Port=7
  terminalPose : Inport  Port=8
  departPose : Inport  Port=9
  w_measure : Inport  Port=10
  resetPose : Inport  Port=11
  Chart : Stateflow chart  TreatAsAtomicUnit=on
  Constant : Constant  Value=0
  Constant1 : Constant  Value=[0;0]
  Constant12 : Constant  Value=0
  Demux : Demux  Outputs=[3,3]
  Demux1 : Demux  Outputs=[2,1]
  Demux3 : Demux  Outputs=3
  Demux4 : Demux  Outputs=[2,1]
  Display : Display
  Forward Kinematics : MATLAB Function  TreatAsAtomicUnit=on
  Integrator : Integrator
  Integrator1 : Integrator  ExternalReset=either  InitialCondition=[0;0;0]
  Integrator4 : Integrator  ExternalReset=either  InitialCondition=[0;0;0]
  Inverse Kinematics1 : MATLAB Function  TreatAsAtomicUnit=on
  MATLAB Function1 : MATLAB Function  TreatAsAtomicUnit=on
  Mux : Mux  Inputs=[3,1,2]
  Mux3 : Mux  Inputs=3
  PID Controller3 : simulink/Continuous/PID Controller  Controller=PID  Form=Parallel  TimeDomain=Continuous-time  SampleTime=-1  IntegratorMethod=Forward Euler  FilterMethod=Forward Euler  ControllerParametersSource=internal  P=5  I=5  D=0  UseFilter=on  N=100  TunerSelectOption=Transfer Function Based (PID Tuner App)  InitialConditionSource=internal  InitialConditionForIntegrator=0  InitialConditionForFilter=0  DifferentiatorICPrevScaledInput=0  ExternalReset=none  TrackingMode=off  Kt=1  LimitOutput=off  UpperSaturationLimit=inf  LowerSaturationLimit=-inf  LinearizeAsGain=on  AntiWindupMode=none  Kb=1  POutMin=[]  POutMax=[]  IOutMin=[]  IOutMax=[]  DOutMin=[]  DOutMax=[]  NOutMin=[]  NOutMax=[]  SumOutMin=[]  SumOutMax=[]  SaturationOutMin=[]  SaturationOutMax=[]  PParamMin=[]  PParamMax=[]  IParamMin=[]  IParamMax=[]  DParamMin=[]  DParamMax=[]  NParamMin=[]  NParamMax=[]  KbParamMin=[]  KbParamMax=[]  KtParamMin=[]  KtParamMax=[]  KbOutMin=[]  KbOutMax=[]  KtOutMin=[]  KtOutMax=[]  IntegratorOutMin=[]  IntegratorOutMax=[]  FilterOutMin=[]  FilterOutMax=[]  SumI1OutMin=[]  SumI1OutMax=[]  SumI2OutMin=[]  SumI2OutMax=[]  SumI3OutMin=[]  SumI3OutMax=[]  SumI4OutMin=[]  SumI4OutMax=[]  SumDOutMin=[]  SumDOutMax=[]  DifferentiatorOutMin=[]  DifferentiatorOutMax=[]  FilterDiffOutCoefMin=[]  FilterDiffOutCoefMax=[]  ReciprocalOutMin=[]  ReciprocalOutMax=[]  SumDenOutMin=[]  SumDenOutMax=[]  SumNumOutMin=[]  SumNumOutMax=[]  DivideOutMin=[]  DivideOutMax=[]  IntegratorContinuousStateAttributes=''  IntegratorStateMustResolveToSignalObject=off  IntegratorRTWStateStorageClass=Auto  FilterContinuousStateAttributes=''  FilterStateMustResolveToSignalObject=off  FilterRTWStateStorageClass=Auto  ParallelPVariant=InternalParameters  IdealPVariant=Disabled  IVariant=InternalParameters  DVariant=InternalParameters  IntegratorVariant=Continuous  SatVariant=Disabled  AWVariant=Passthrough  PCopyVariant=Disabled  TRVariant=Disabled  FdbkBlocksVariant=Forward  IdealPFdbkVariant=Disabled  SatFdbkVariant=Disabled  DerivativeFilterVariant=ContFilter  NVariant=InternalParameters  NCopyVariant=Disabled  FilterICVariant=InternalICsFilter  IntegratorICVariant=InternalICs  ExternalResetVariant=Disabled  TRSumVariant=Passthrough  SumFdbkVariant=Disabled  SumVariant=Sum_PID
  PID Controller4 : simulink/Continuous/PID Controller  Controller=PID  Form=Parallel  TimeDomain=Continuous-time  SampleTime=-1  IntegratorMethod=Forward Euler  FilterMethod=Forward Euler  ControllerParametersSource=internal  P=5  I=5  D=0  UseFilter=on  N=100  TunerSelectOption=Transfer Function Based (PID Tuner App)  InitialConditionSource=internal  InitialConditionForIntegrator=0  InitialConditionForFilter=0  DifferentiatorICPrevScaledInput=0  ExternalReset=none  TrackingMode=off  Kt=1  LimitOutput=off  UpperSaturationLimit=inf  LowerSaturationLimit=-inf  LinearizeAsGain=on  AntiWindupMode=none  Kb=1  POutMin=[]  POutMax=[]  IOutMin=[]  IOutMax=[]  DOutMin=[]  DOutMax=[]  NOutMin=[]  NOutMax=[]  SumOutMin=[]  SumOutMax=[]  SaturationOutMin=[]  SaturationOutMax=[]  PParamMin=[]  PParamMax=[]  IParamMin=[]  IParamMax=[]  DParamMin=[]  DParamMax=[]  NParamMin=[]  NParamMax=[]  KbParamMin=[]  KbParamMax=[]  KtParamMin=[]  KtParamMax=[]  KbOutMin=[]  KbOutMax=[]  KtOutMin=[]  KtOutMax=[]  IntegratorOutMin=[]  IntegratorOutMax=[]  FilterOutMin=[]  FilterOutMax=[]  SumI1OutMin=[]  SumI1OutMax=[]  SumI2OutMin=[]  SumI2OutMax=[]  SumI3OutMin=[]  SumI3OutMax=[]  SumI4OutMin=[]  SumI4OutMax=[]  SumDOutMin=[]  SumDOutMax=[]  DifferentiatorOutMin=[]  DifferentiatorOutMax=[]  FilterDiffOutCoefMin=[]  FilterDiffOutCoefMax=[]  ReciprocalOutMin=[]  ReciprocalOutMax=[]  SumDenOutMin=[]  SumDenOutMax=[]  SumNumOutMin=[]  SumNumOutMax=[]  DivideOutMin=[]  DivideOutMax=[]  IntegratorContinuousStateAttributes=''  IntegratorStateMustResolveToSignalObject=off  IntegratorRTWStateStorageClass=Auto  FilterContinuousStateAttributes=''  FilterStateMustResolveToSignalObject=off  FilterRTWStateStorageClass=Auto  ParallelPVariant=InternalParameters  IdealPVariant=Disabled  IVariant=InternalParameters  DVariant=InternalParameters  IntegratorVariant=Continuous  SatVariant=Disabled  AWVariant=Passthrough  PCopyVariant=Disabled  TRVariant=Disabled  FdbkBlocksVariant=Forward  IdealPFdbkVariant=Disabled  SatFdbkVariant=Disabled  DerivativeFilterVariant=ContFilter  NVariant=InternalParameters  NCopyVariant=Disabled  FilterICVariant=InternalICsFilter  IntegratorICVariant=InternalICs  ExternalResetVariant=Disabled  TRSumVariant=Passthrough  SumFdbkVariant=Disabled  SumVariant=Sum_PID
  PID Controller5 : simulink/Continuous/PID Controller  Controller=PID  Form=Parallel  TimeDomain=Continuous-time  SampleTime=-1  IntegratorMethod=Forward Euler  FilterMethod=Forward Euler  ControllerParametersSource=internal  P=5  I=5  D=0  UseFilter=on  N=100  TunerSelectOption=Transfer Function Based (PID Tuner App)  InitialConditionSource=internal  InitialConditionForIntegrator=0  InitialConditionForFilter=0  DifferentiatorICPrevScaledInput=0  ExternalReset=none  TrackingMode=off  Kt=1  LimitOutput=off  UpperSaturationLimit=inf  LowerSaturationLimit=-inf  LinearizeAsGain=on  AntiWindupMode=none  Kb=1  POutMin=[]  POutMax=[]  IOutMin=[]  IOutMax=[]  DOutMin=[]  DOutMax=[]  NOutMin=[]  NOutMax=[]  SumOutMin=[]  SumOutMax=[]  SaturationOutMin=[]  SaturationOutMax=[]  PParamMin=[]  PParamMax=[]  IParamMin=[]  IParamMax=[]  DParamMin=[]  DParamMax=[]  NParamMin=[]  NParamMax=[]  KbParamMin=[]  KbParamMax=[]  KtParamMin=[]  KtParamMax=[]  KbOutMin=[]  KbOutMax=[]  KtOutMin=[]  KtOutMax=[]  IntegratorOutMin=[]  IntegratorOutMax=[]  FilterOutMin=[]  FilterOutMax=[]  SumI1OutMin=[]  SumI1OutMax=[]  SumI2OutMin=[]  SumI2OutMax=[]  SumI3OutMin=[]  SumI3OutMax=[]  SumI4OutMin=[]  SumI4OutMax=[]  SumDOutMin=[]  SumDOutMax=[]  DifferentiatorOutMin=[]  DifferentiatorOutMax=[]  FilterDiffOutCoefMin=[]  FilterDiffOutCoefMax=[]  ReciprocalOutMin=[]  ReciprocalOutMax=[]  SumDenOutMin=[]  SumDenOutMax=[]  SumNumOutMin=[]  SumNumOutMax=[]  DivideOutMin=[]  DivideOutMax=[]  IntegratorContinuousStateAttributes=''  IntegratorStateMustResolveToSignalObject=off  IntegratorRTWStateStorageClass=Auto  FilterContinuousStateAttributes=''  FilterStateMustResolveToSignalObject=off  FilterRTWStateStorageClass=Auto  ParallelPVariant=InternalParameters  IdealPVariant=Disabled  IVariant=InternalParameters  DVariant=InternalParameters  IntegratorVariant=Continuous  SatVariant=Disabled  AWVariant=Passthrough  PCopyVariant=Disabled  TRVariant=Disabled  FdbkBlocksVariant=Forward  IdealPFdbkVariant=Disabled  SatFdbkVariant=Disabled  DerivativeFilterVariant=ContFilter  NVariant=InternalParameters  NCopyVariant=Disabled  FilterICVariant=InternalICsFilter  IntegratorICVariant=InternalICs  ExternalResetVariant=Disabled  TRSumVariant=Passthrough  SumFdbkVariant=Disabled  SumVariant=Sum_PID
  Rotation Matrix (R(theta)) : MATLAB Function  TreatAsAtomicUnit=on
  Scope : Scope
  Scope1 : Scope
  Scope2 : Scope
  Sum1 : Sum  Inputs=++|
  Sum2 : Sum  Inputs=|+-
  Switch2 : Switch  Criteria=u2 ~= 0
  Switch3 : Switch  Criteria=u2 ~= 0
  Terminator2 : Terminator
  Terminator3 : Terminator
  Terminator4 : Terminator
  Trajectory velocity generation : MATLAB Function  TreatAsAtomicUnit=on
  UDP receive : Constant  Value=0
  fi_dot : Outport
  robotPose : Outport  Port=2
  desiredVel : Outport  Port=3
  desiredPose : Outport  Port=4
  wires:
  Demux3/2 -> PID Controller4/1
  Rotation Matrix (R(theta))/1(X_w_dot) -> Integrator4/1
  manual/1 -> Switch3/2, Switch2/2
  PID Controller3/1 -> Mux3/1
  Constant/1 -> Switch2/1
  Trajectory velocity generation/1(X_r_dot) -> desiredVel/1, Sum1/1, Integrator1/1
  Sum1/1 -> Inverse Kinematics1/2(u)
  Integrator1/1 -> desiredPose/1, Demux1/1, Scope1/1, Sum2/1
  Mux3/1 -> Sum1/2
  Demux3/3 -> PID Controller5/1
  Demux1/1 -> Terminator3/1
  Forward Kinematics/1(x_dot) -> Rotation Matrix (R(theta))/2(X_R_dot)
  Integrator4/1 -> robotPose/1, Sum2/2, Demux4/1
  t_dep/1 -> Trajectory velocity generation/2(t_dep)
  Inverse Kinematics1/1(fi_dot) -> Scope2/1, Mux/1
  accel/1 -> Trajectory velocity generation/4(accel)
  PID Controller4/1 -> Mux3/2
  Demux4/1 -> Terminator2/1
  Demux4/2 -> Switch3/3
  PID Controller5/1 -> Mux3/3
  Demux3/1 -> PID Controller3/1
  Switch2/1 -> Inverse Kinematics1/1(thetad)
  Switch3/1 -> Rotation Matrix (R(theta))/1(theta)
  Demux1/2 -> Switch2/3
  t/1 -> [t], Trajectory velocity generation/1(t)
  Constant12/1 -> Switch3/1
  Demux/1 -> Forward Kinematics/1(fi_dot)
  Vmax/1 -> Trajectory velocity generation/3(Vmax)
  terminalPose/1 -> Trajectory velocity generation/7(terminalPose)
  omegaMax/1 -> Trajectory velocity generation/5(omegaMax)
  angAccel/1 -> Trajectory velocity generation/6(angAccel)
  departPose/1 -> Trajectory velocity generation/8(departPose)
  Mux/1 -> fi_dot/1
  MATLAB Function1/2(omega) -> Integrator/1, Mux/2
  w_measure/1 -> Demux/1
  resetPose/1 -> Integrator1/2, Integrator4/2
  [t] -> MATLAB Function1/1(t)
  Constant1/1 -> Mux/3
  UDP receive/1 -> Chart/2(kick)
  Integrator/1 -> Chart/3(theta_d)
  Chart/4(departPose) -> MATLAB Function1/5(departPose)
  Chart/1(t_dep) -> MATLAB Function1/2(t_dep)
  Chart/2(omegaMax) -> MATLAB Function1/3(omegaMax)
  Chart/3(terminalPose) -> MATLAB Function1/4(terminalPose)
  MATLAB Function1/1(Ts) -> Display/1
  Sum2/1 -> Scope/1, Demux3/1
  Demux/2 -> Terminator4/1

== system full_3omni_ctrl_sim_and_exp_with_bbb/Sending Robot Location to Smart Phone ==
  robotPose : Inport
  Demux2 : Demux  Outputs=3
  Logical Operator4 : Logic  Operator=NOT  AllPortsSameDT=off  OutDataTypeStr=boolean
  Logical Operator5 : Logic  AllPortsSameDT=off  OutDataTypeStr=boolean
  Pulse Generator : DiscretePulseGenerator  PulseType=Time based  Period=5  PulseWidth=50
  Sending Location of Robot : Subsystem
  Unit Delay2 : UnitDelay  SampleTime=-1  HasFrameUpgradeWarning=on
  wires:
  Demux2/3 -> Sending Location of Robot/3(z)
  Demux2/2 -> Sending Location of Robot/2(y)
  Demux2/1 -> Sending Location of Robot/1(x)
  Logical Operator5/1 -> Sending Location of Robot/Enable
  robotPose/1 -> Demux2/1
  Pulse Generator/1 -> Logical Operator5/1, Unit Delay2/1
  Unit Delay2/1 -> Logical Operator4/1
  Logical Operator4/1 -> Logical Operator5/2

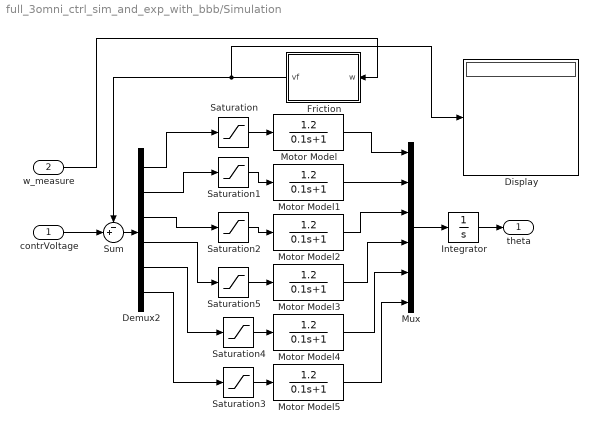
== system full_3omni_ctrl_sim_and_exp_with_bbb/Simulation ==
  contrVoltage : Inport
  w_measure : Inport  Port=2
  Demux2 : Demux  Outputs=6
  Display : Display
  Friction : MATLAB Function  TreatAsAtomicUnit=on
  Integrator : Integrator  InitialCondition=zeros(6,1)
  Motor Model{,1..5} (6 alike) : TransferFcn  Numerator=[1.2]  Denominator=[0.1 1]
  Mux : Mux  Inputs=6
  Saturation{,1..5} (6 alike) : Saturate  UpperLimit=19  LowerLimit=-19
  Sum : Sum  Inputs=-+|
  theta : Outport
  wires:
  contrVoltage/1 -> Sum/2
  Demux2/1 -> Saturation/1
  Motor Model2/1 -> Mux/3
  Motor Model3/1 -> Mux/4
  Motor Model4/1 -> Mux/5
  Motor Model5/1 -> Mux/6
  Demux2/2 -> Saturation1/1
  Demux2/3 -> Saturation2/1
  Demux2/4 -> Saturation5/1
  Demux2/5 -> Saturation4/1
  Demux2/6 -> Saturation3/1
  Mux/1 -> Integrator/1
  Friction/1(vf) -> Display/1, Sum/1
  Sum/1 -> Demux2/1
  w_measure/1 -> Friction/1(w)
  Integrator/1 -> theta/1
  Motor Model/1 -> Mux/1
  Motor Model1/1 -> Mux/2
  Saturation/1 -> Motor Model/1
  Saturation1/1 -> Motor Model1/1
  Saturation2/1 -> Motor Model2/1
  Saturation3/1 -> Motor Model5/1
  Saturation4/1 -> Motor Model4/1
  Saturation5/1 -> Motor Model3/1

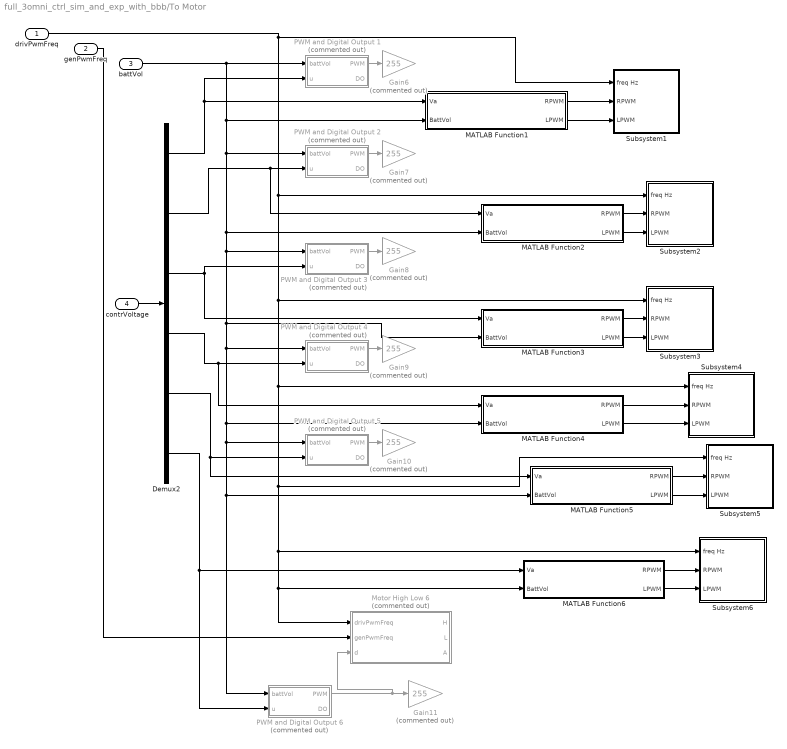
== system full_3omni_ctrl_sim_and_exp_with_bbb/To Motor ==
  drivPwmFreq : Inport
  genPwmFreq : Inport  Port=2
  battVol : Inport  Port=3
  contrVoltage : Inport  Port=4
  Demux2 : Demux  Outputs=6
  Gain{6..11} (6 alike) : Gain  Commented=on  Gain=255
  MATLAB Function1 : MATLAB Function  TreatAsAtomicUnit=on
  MATLAB Function2 : MATLAB Function  TreatAsAtomicUnit=on
  MATLAB Function3 : MATLAB Function  TreatAsAtomicUnit=on
  MATLAB Function4 : MATLAB Function  TreatAsAtomicUnit=on
  MATLAB Function5 : MATLAB Function  TreatAsAtomicUnit=on
  MATLAB Function6 : MATLAB Function  TreatAsAtomicUnit=on
  Motor High Low 6 : MATLAB Function  Commented=on  TreatAsAtomicUnit=on
  PWM and Digital Output 1 : MATLAB Function  Commented=on  TreatAsAtomicUnit=on
  PWM and Digital Output 2 : MATLAB Function  Commented=on  TreatAsAtomicUnit=on
  PWM and Digital Output 3 : MATLAB Function  Commented=on  TreatAsAtomicUnit=on
  PWM and Digital Output 4 : MATLAB Function  Commented=on  TreatAsAtomicUnit=on
  PWM and Digital Output 5 : MATLAB Function  Commented=on  TreatAsAtomicUnit=on
  PWM and Digital Output 6 : MATLAB Function  Commented=on  TreatAsAtomicUnit=on
  Subsystem1 : Subsystem
  Subsystem2 : Subsystem
  Subsystem3 : Subsystem
  Subsystem4 : Subsystem
  Subsystem5 : Subsystem
  Subsystem6 : Subsystem
  wires:
  PWM and Digital Output 6/1(PWM) -> Motor High Low 6/3(d), Gain11/1
  genPwmFreq/1 -> Motor High Low 6/2(genPwmFreq)
  Demux2/4 -> MATLAB Function4/1(Va), PWM and Digital Output 4/2(u)
  Demux2/5 -> MATLAB Function5/1(Va), PWM and Digital Output 5/2(u)
  PWM and Digital Output 4/1(PWM) -> Gain9/1
  Demux2/2 -> MATLAB Function2/1(Va), PWM and Digital Output 2/2(u)
  Demux2/3 -> MATLAB Function3/1(Va), PWM and Digital Output 3/2(u)
  Demux2/6 -> MATLAB Function6/1(Va), PWM and Digital Output 6/2(u)
  contrVoltage/1 -> Demux2/1
  PWM and Digital Output 3/1(PWM) -> Gain8/1
  PWM and Digital Output 1/1(PWM) -> Gain6/1
  PWM and Digital Output 5/1(PWM) -> Gain10/1
  PWM and Digital Output 2/1(PWM) -> Gain7/1
  Demux2/1 -> PWM and Digital Output 1/2(u), MATLAB Function1/1(Va)
  MATLAB Function1/2(LPWM) -> Subsystem1/3(LPWM)
  MATLAB Function1/1(RPWM) -> Subsystem1/2(RPWM)
  battVol/1 -> PWM and Digital Output 2/1(battVol), MATLAB Function2/2(BattVol), PWM and Digital Output 3/1(battVol), MATLAB Function3/2(BattVol), PWM and Digital Output 4/1(battVol), MATLAB Function4/2(BattVol), PWM and Digital Output 5/1(battVol), PWM and Digital Output 6/1(battVol), MATLAB Function5/2(BattVol), MATLAB Function1/2(BattVol), PWM and Digital Output 1/1(battVol)
  MATLAB Function2/1(RPWM) -> Subsystem2/2(RPWM)
  MATLAB Function2/2(LPWM) -> Subsystem2/3(LPWM)
  drivPwmFreq/1 -> Subsystem2/1(freq Hz), Subsystem3/1(freq Hz), Subsystem6/1(freq Hz), MATLAB Function6/2(BattVol), Motor High Low 6/1(drivPwmFreq), Subsystem5/1(freq Hz), Subsystem4/1(freq Hz), Subsystem1/1(freq Hz)
  MATLAB Function3/1(RPWM) -> Subsystem3/2(RPWM)
  MATLAB Function3/2(LPWM) -> Subsystem3/3(LPWM)
  MATLAB Function4/1(RPWM) -> Subsystem4/2(RPWM)
  MATLAB Function4/2(LPWM) -> Subsystem4/3(LPWM)
  MATLAB Function5/2(LPWM) -> Subsystem5/3(LPWM)
  MATLAB Function5/1(RPWM) -> Subsystem5/2(RPWM)
  MATLAB Function6/2(LPWM) -> Subsystem6/3(LPWM)
  MATLAB Function6/1(RPWM) -> Subsystem6/2(RPWM)

== system full_3omni_ctrl_sim_and_exp_with_bbb/Sending Robot Location to Smart Phone/Sending Location of Robot ==
  x : Inport
  y : Inport  Port=2
  z : Inport  Port=3
  Enable : EnablePort
  "Byte Packing " : xpcutilitieslib/Byte Packing   MaskPackedDataType=uint8  MaskUnpackedDataTypes={'double'}  MaskAlignment=1
  Display1 : Display
  Mux : Mux  Inputs=3
  "Send " : slrtlib/UDP/Send   localPort=-1  ipAddress=192.168.88.233  ipPort=2500  sampletime=-1
      settings: SourceProductName=Simulink Real-Time  SourceProductBaseCode=XP
  wires:
  "Byte Packing "/1 -> "Send "/1
  Mux/1 -> Display1/1, "Byte Packing "/1
  y/1 -> Mux/2
  z/1 -> Mux/3
  x/1 -> Mux/1

== system full_3omni_ctrl_sim_and_exp_with_bbb/To Motor/Subsystem1 ==
  freq Hz : Inport
  RPWM : Inport  Port=2
  LPWM : Inport  Port=3
  Constant1 : Constant  Value=0
  Generate PWM : Subsystem
  NOT : Logic  Operator=NOT  IconShape=distinctive  AllPortsSameDT=off  OutDataTypeStr=boolean
  Setup : Subsystem
  Unit Delay : UnitDelay  InitialCondition=1  SampleTime=-1  HasFrameUpgradeWarning=on
  wires:
  Constant1/1 -> Unit Delay/1
  NOT/1 -> Generate PWM/Enable
  Unit Delay/1 -> Setup/Enable, NOT/1
  freq Hz/1 -> Setup/1(freq Hz)
  RPWM/1 -> Generate PWM/1(RPWM)
  LPWM/1 -> Generate PWM/2(LPWM)

== system full_3omni_ctrl_sim_and_exp_with_bbb/To Motor/Subsystem2 ==
  freq Hz : Inport
  RPWM : Inport  Port=2
  LPWM : Inport  Port=3
  Constant1 : Constant  Value=0
  Generate PWM : Subsystem
  NOT : Logic  Operator=NOT  IconShape=distinctive  AllPortsSameDT=off  OutDataTypeStr=boolean
  Setup : Subsystem  Commented=on
  Unit Delay : UnitDelay  InitialCondition=1  SampleTime=-1  HasFrameUpgradeWarning=on
  wires:
  Constant1/1 -> Unit Delay/1
  NOT/1 -> Generate PWM/Enable
  Unit Delay/1 -> Setup/Enable, NOT/1
  freq Hz/1 -> Setup/1(freq Hz)
  RPWM/1 -> Generate PWM/1(RPWM)
  LPWM/1 -> Generate PWM/2(LPWM)

== system full_3omni_ctrl_sim_and_exp_with_bbb/To Motor/Subsystem3 ==
  freq Hz : Inport
  RPWM : Inport  Port=2
  LPWM : Inport  Port=3
  Constant1 : Constant  Value=0
  Generate PWM : Subsystem
  NOT : Logic  Operator=NOT  IconShape=distinctive  AllPortsSameDT=off  OutDataTypeStr=boolean
  Setup : Subsystem  Commented=on
  Unit Delay : UnitDelay  InitialCondition=1  SampleTime=-1  HasFrameUpgradeWarning=on
  wires:
  Constant1/1 -> Unit Delay/1
  NOT/1 -> Generate PWM/Enable
  Unit Delay/1 -> Setup/Enable, NOT/1
  freq Hz/1 -> Setup/1(freq Hz)
  RPWM/1 -> Generate PWM/1(RPWM)
  LPWM/1 -> Generate PWM/2(LPWM)

== system full_3omni_ctrl_sim_and_exp_with_bbb/To Motor/Subsystem4 ==
  freq Hz : Inport
  RPWM : Inport  Port=2
  LPWM : Inport  Port=3
  Constant1 : Constant  Value=0
  Generate PWM : Subsystem
  NOT : Logic  Operator=NOT  IconShape=distinctive  AllPortsSameDT=off  OutDataTypeStr=boolean
  Setup : Subsystem  Commented=on
  Unit Delay : UnitDelay  InitialCondition=1  SampleTime=-1  HasFrameUpgradeWarning=on
  wires:
  Constant1/1 -> Unit Delay/1
  NOT/1 -> Generate PWM/Enable
  Unit Delay/1 -> Setup/Enable, NOT/1
  freq Hz/1 -> Setup/1(freq Hz)
  RPWM/1 -> Generate PWM/1(RPWM)
  LPWM/1 -> Generate PWM/2(LPWM)

== system full_3omni_ctrl_sim_and_exp_with_bbb/To Motor/Subsystem5 ==
  freq Hz : Inport
  RPWM : Inport  Port=2
  LPWM : Inport  Port=3
  Constant1 : Constant  Value=0
  Generate PWM : Subsystem
  NOT : Logic  Operator=NOT  IconShape=distinctive  AllPortsSameDT=off  OutDataTypeStr=boolean
  Setup : Subsystem  Commented=on
  Unit Delay : UnitDelay  InitialCondition=1  SampleTime=-1  HasFrameUpgradeWarning=on
  wires:
  Constant1/1 -> Unit Delay/1
  NOT/1 -> Generate PWM/Enable
  Unit Delay/1 -> Setup/Enable, NOT/1
  freq Hz/1 -> Setup/1(freq Hz)
  RPWM/1 -> Generate PWM/1(RPWM)
  LPWM/1 -> Generate PWM/2(LPWM)

== system full_3omni_ctrl_sim_and_exp_with_bbb/To Motor/Subsystem6 ==
  freq Hz : Inport
  RPWM : Inport  Port=2
  LPWM : Inport  Port=3
  Constant1 : Constant  Value=0
  Generate PWM : Subsystem
  NOT : Logic  Operator=NOT  IconShape=distinctive  AllPortsSameDT=off  OutDataTypeStr=boolean
  Setup : Subsystem  Commented=on
  Unit Delay : UnitDelay  InitialCondition=1  SampleTime=-1  HasFrameUpgradeWarning=on
  wires:
  Constant1/1 -> Unit Delay/1
  NOT/1 -> Generate PWM/Enable
  Unit Delay/1 -> Setup/Enable, NOT/1
  freq Hz/1 -> Setup/1(freq Hz)
  RPWM/1 -> Generate PWM/1(RPWM)
  LPWM/1 -> Generate PWM/2(LPWM)
